simulink model "Longitudinal_Vehicle_Model"  (R2016b)
settings: Solver=ode3  StartTime=0.0  StopTime=1500  FixedStep=0.001  RelTol=1e-3
InitFcn:
  | % Call parameters initialization function
  | % run optiTruck_init_sim.m;
StopFcn:
  | %optiTruck_post_sim;
  | %optiTruck_plot_sim;
undefined symbols (not defined in the file or in its folder): DiscIntNeverNeededParam
settings Model: Creator=engin  LastModifiedBy=engin.ozatay
settings DataIOCC: SaveFormat=StructureWithTime  SaveOutput=off  SaveTime=off
settings OptimizationCC: BlockReduction=off  BufferReuse=off  LifeSpan=inf
settings DebuggingCC: AlgebraicLoopMsg=none  UnconnectedInputMsg=none  UnconnectedOutputMsg=none  UnconnectedLineMsg=none  SFExecutionAtInitializationDiag=none
settings HardwareCC: ProdBitPerSizeT=32  ProdBitPerPtrDiffT=32  ProdWordSize=32  ProdHWDeviceType=Specified

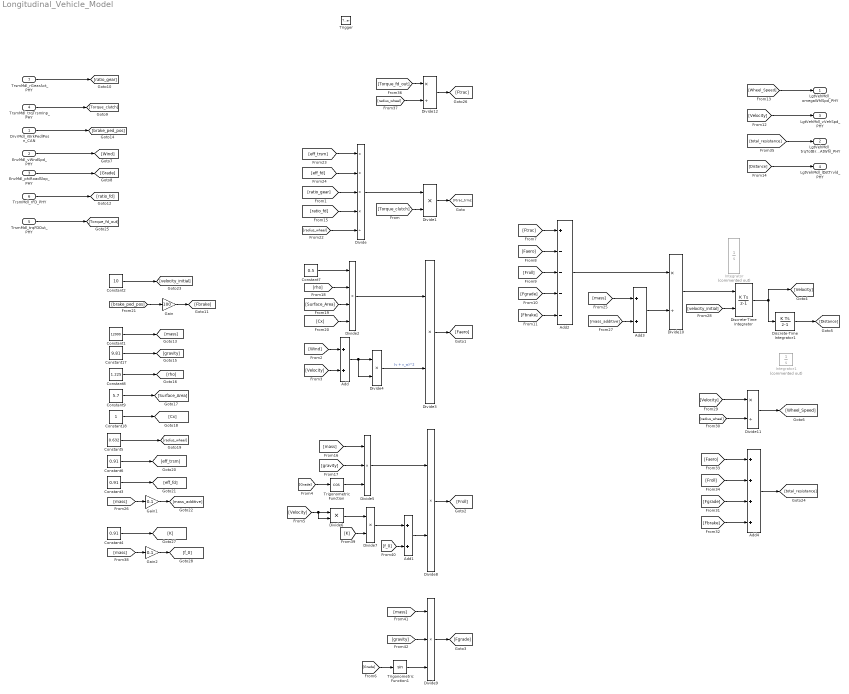
== system Longitudinal_Vehicle_Model ==
  DrvrMdl_rBrkPedlPosn_CAN : Inport
  EnvMdl_vWndSpd_PHY : Inport  Port=2
  EnvMdl_phiRoadSlop_PHY : Inport  Port=3
  TrsmMdl_trqTrsmInp_PHY : Inport  Port=4
  TrsmMdl_trqFDOut_PHY : Inport  Port=5
  TrsmMdl_rFD_PHY : Inport  Port=6
  TrsmMdl_rGearAct_PHY : Inport  Port=7
  Trigger : TriggerPort  TriggerType=function-call  VariantControl=Variant  PortDimensions=1
  Add : Sum
  Add1 : Sum
  Add2 : Sum  Inputs=+----
  Add3 : Sum
  Add4 : Sum  Inputs=++++
  Constant1 : Constant  Value=12000  SampleTime=-1
  Constant17 : Constant  Value=9.81  SampleTime=-1
  Constant18 : Constant  SampleTime=-1
  Constant2 : Constant  Value=10  SampleTime=-1
  Constant3 : Constant  Value=0.91  SampleTime=-1
  Constant4 : Constant  Value=0.91  SampleTime=-1
  Constant5 : Constant  Value=0.632  SampleTime=-1
  Constant6 : Constant  Value=0.91  SampleTime=-1
  Constant7 : Constant  Value=0.5  SampleTime=-1
  Constant8 : Constant  Value=1.225  SampleTime=-1
  Constant9 : Constant  Value=5.7  SampleTime=-1
  Discrete-Time Integrator : DiscreteIntegrator  InitialConditionSource=external  SampleTime=-1  ICPrevOutput=DiscIntNeverNeededParam  ICPrevScaledInput=DiscIntNeverNeededParam
  Discrete-Time Integrator1 : DiscreteIntegrator  SampleTime=-1  ICPrevOutput=DiscIntNeverNeededParam  ICPrevScaledInput=DiscIntNeverNeededParam
  Divide : Product  Inputs=****/
  Divide{1,3..4,6..8} (6 alike) : Product  Inputs=**
  Divide10 : Product  Inputs=*/
  Divide11 : Product  Inputs=*/
  Divide12 : Product  Inputs=*/
  Divide2 : Product  Inputs=****
  Divide5 : Product  Inputs=***
  Divide9 : Product  Inputs=***
  Gain : Gain  Gain=100
  Gain1 : Gain  Gain=0.1
  Gain2 : Gain  Gain=0.1
  Integrator : Integrator  Commented=on  InitialConditionSource=external
  Integrator1 : Integrator  Commented=on
  Trigonometric Function : Trigonometry  Operator=cos
  Trigonometric Function1 : Trigonometry
  LgtVehMdl_omegaWhlSpd_PHY : Outport
  LgtVehMdl_trqTotBrkRAtWhl_PHY : Outport  Port=2
  LgtVehMdl_vVehSpd_PHY : Outport  Port=3
  LgtVehMdl_lDstTrvld_PHY : Outport  Port=4
  wires:
  [Velocity] -> LgtVehMdl_vVehSpd_PHY/1
  [Wheel_Speed] -> LgtVehMdl_omegaWhlSpd_PHY/1
  [total_resistance] -> LgtVehMdl_trqTotBrkRAtWhl_PHY/1
  EnvMdl_vWndSpd_PHY/1 -> [Wind]
  EnvMdl_phiRoadSlop_PHY/1 -> [Grade]
  [eff_fd] -> Divide/2
  [Torque_clutch] -> Divide1/2
  [ratio_gear] -> Divide/3
  Divide/1 -> Divide1/1
  Divide1/1 -> [Ftrac_trms]
  [eff_trsm] -> Divide/1
  Add/1 -> Divide4/1, Divide4/2
  Divide3/1 -> [Faero]
  [Wind] -> Add/1
  [rho] -> Divide2/2
  [Surface_Area] -> Divide2/3
  Constant7/1 -> Divide2/1
  Divide2/1 -> Divide3/1
  [Velocity] -> Add/2
  [Cx] -> Divide2/4
  Divide4/1 -> Divide3/2  "(v + v_w)^2"
  [gravity] -> Divide5/2
  Add1/1 -> Divide8/2
  Divide7/1 -> Add1/1
  [mass] -> Divide5/1
  [K] -> Divide7/2
  Divide6/1 -> Divide7/1
  Divide5/1 -> Divide8/1
  [Grade] -> Trigonometric Function/1
  [f_0] -> Add1/2
  Trigonometric Function/1 -> Divide5/3
  [Velocity] -> Divide6/1, Divide6/2
  Divide8/1 -> [Froll]
  Trigonometric Function1/1 -> Divide9/3
  Divide9/1 -> [Fgrade]
  [Grade] -> Trigonometric Function1/1
  [velocity_initial] -> Discrete-Time Integrator/2
  [Froll] -> Add2/3
  [Fbrake] -> Add2/5
  Add2/1 -> Divide10/1
  [mass_additive] -> Add3/2
  [mass] -> Add3/1
  [Fgrade] -> Add2/4
  Add3/1 -> Divide10/2
  [Faero] -> Add2/2
  [Ftrac] -> Add2/1
  TrsmMdl_trqTrsmInp_PHY/1 -> [Torque_clutch]
  TrsmMdl_rGearAct_PHY/1 -> [ratio_gear]
  [Distance] -> LgtVehMdl_lDstTrvld_PHY/1
  [radius_wheel] -> Divide/5
  [ratio_fd] -> Divide/4
  TrsmMdl_rFD_PHY/1 -> [ratio_fd]
  Constant1/1 -> [mass]
  DrvrMdl_rBrkPedlPosn_CAN/1 -> [brake_ped_pos]
  Constant17/1 -> [gravity]
  Constant8/1 -> [rho]
  Constant9/1 -> [Surface_Area]
  Constant18/1 -> [Cx]
  [brake_ped_pos] -> Gain/1
  Gain/1 -> [Fbrake]
  Constant5/1 -> [radius_wheel]
  Constant6/1 -> [eff_trsm]
  Constant3/1 -> [eff_fd]
  [mass] -> Gain1/1
  Gain1/1 -> [mass_additive]
  Constant2/1 -> [velocity_initial]
  Divide11/1 -> [Wheel_Speed]
  [Velocity] -> Divide11/1
  [radius_wheel] -> Divide11/2
  [Faero] -> Add4/1
  [Froll] -> Add4/2
  [Fgrade] -> Add4/3
  [Fbrake] -> Add4/4
  Add4/1 -> [total_resistance]
  [radius_wheel] -> Divide12/2
  [Torque_fd_out] -> Divide12/1
  Divide12/1 -> [Ftrac]
  TrsmMdl_trqFDOut_PHY/1 -> [Torque_fd_out]
  Constant4/1 -> [K]
  [mass] -> Gain2/1
  Gain2/1 -> [f_0]
  [gravity] -> Divide9/2
  [mass] -> Divide9/1
  Discrete-Time Integrator1/1 -> [Distance]
  Discrete-Time Integrator/1 -> [Velocity], Discrete-Time Integrator1/1
  Divide10/1 -> Discrete-Time Integrator/1
